simulink model "EPD629_WilliamsJ_Project_20220413_1405"  (R2021b)
settings: Solver=VariableStepAuto  StartTime=0.0  StopTime=25  MaxStep=0.005  RelTol=1e-3
values from neighbouring files (symbols this model uses):
  AxleRatio = 11.47    [ProjectScript.m]
  BrakeDrag_N = 2.5    [ProjectScript.m]
  CableStrokeVsPedalPos_mmpdeg = 0.995519    [ProjectScript.m]
  Cd = 0.7691142    [ProjectScript.m]
  Crr = 0.0138796    [ProjectScript.m]
  CTireRollRadius = 0.944    [ProjectScript.m]
  CVTEff = 0.35    [ProjectScript.m]
  CVTEngagementSpd_rpm = 1400    [ProjectScript.m]
  CVTRatioCoeffVsMphA = 0.000494471902965804    (= 0.000494471902966)    [ProjectScript.m]
  CVTRatioCoeffVsMphB = -0.0203171948865201    (= -0.0203171948865)    [ProjectScript.m]
  CVTRatioCoeffVsMphC = 0.301637634575451    (= 0.301637634575)    [ProjectScript.m]
  CVTRatioCoeffVsMphD = -2.09463337350964    (= -2.09463337351)    [ProjectScript.m]
  CVTRatioCoeffVsMphE = 7.47628950179633    (= 7.4762895018)    [ProjectScript.m]
  DistCableSinkThrottle_mm = 0.25    [ProjectScript.m]
  EngPowerTableData_hp = [0, 0, 0, 0, 0 ... (first row only)    [ProjectScript.m]
  EngPowerTableSpdBreakpoints_rpm = (0:500:7500)    [ProjectScript.m]
  EngPowerTableThrottleBreakpoints_prcnt = [0:.25:1]    [ProjectScript.m]
  FlyCoeffAClosed = 5.31512605042017e-8    (= 5.31512605042e-08)    [ProjectScript.m]
  FlyCoeffAOpen = 2.27450980392157e-7    (= 2.27450980392e-07)    [ProjectScript.m]
  FlyCoeffBClosed = 0.0000162815126050419    (= 1.6281512605e-05)    [ProjectScript.m]
  FlyCoeffBOpen = -0.000070868347338936    (= -7.08683473389e-05)    [ProjectScript.m]
  FlyCoeffCClosed = -0.0102941176470588    (= -0.0102941176471)    [ProjectScript.m]
  FlyCoeffCOpen = 0.00588235294117689    (= 0.00588235294118)    [ProjectScript.m]
  g = 9.80665    [ProjectScript.m]
  GearboxRatio = 1.95    [ProjectScript.m]
  GovArmRange_deg = 14.7    [ProjectScript.m]
  GradeIncline_pcnt = 0    [ProjectScript.m]
  LengthGovArmLower_mm = 90.4    [ProjectScript.m]
  LengthGovArmUpper_mm = 67.5    [ProjectScript.m]
  MassVehicle_kg = (CurbWeight_lbm + VehiclePayload_lbm)*0.4535924    (= 589.67012)    [ProjectScript.m]
  PedalPosMax_deg = 30    [ProjectScript.m]
  PedalTravelIntTension_deg = 10    [ProjectScript.m]
  rho_air = 1.224991    [ProjectScript.m]
  SpringRate_lbfpin = 12.6    [ProjectScript.m]
  ThrottleCableDia_mm = 1.190625    [ProjectScript.m]
  ThrottleLeverArmRadius_mm = 14.25    [ProjectScript.m]
  ThrottlePosMax_deg = 82    [ProjectScript.m]
  ThrottleReturnSpringPreload_Nmm = 163.7711    [ProjectScript.m]
  ThrottleReturnSpringRate_Nmmpdeg = 0.786881    [ProjectScript.m]
  TireDia_in = 18    [ProjectScript.m]
  VehicleFrontalArea_m2 = 1.8    [ProjectScript.m]
libraries: simulink_extras x2
settings Model: Creator=jwilli42  LastModifiedBy=jwilli42

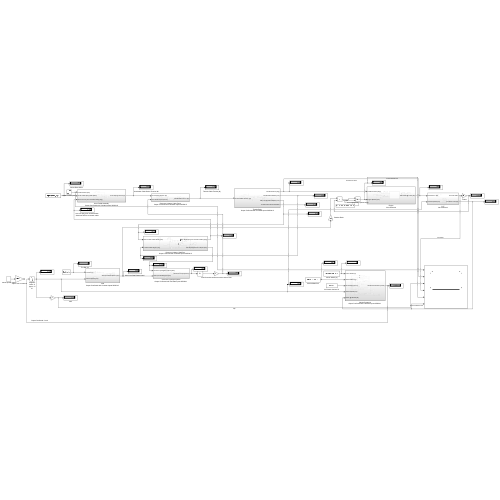
[thumbnail: Simulink's stored preview of the top-level diagram]
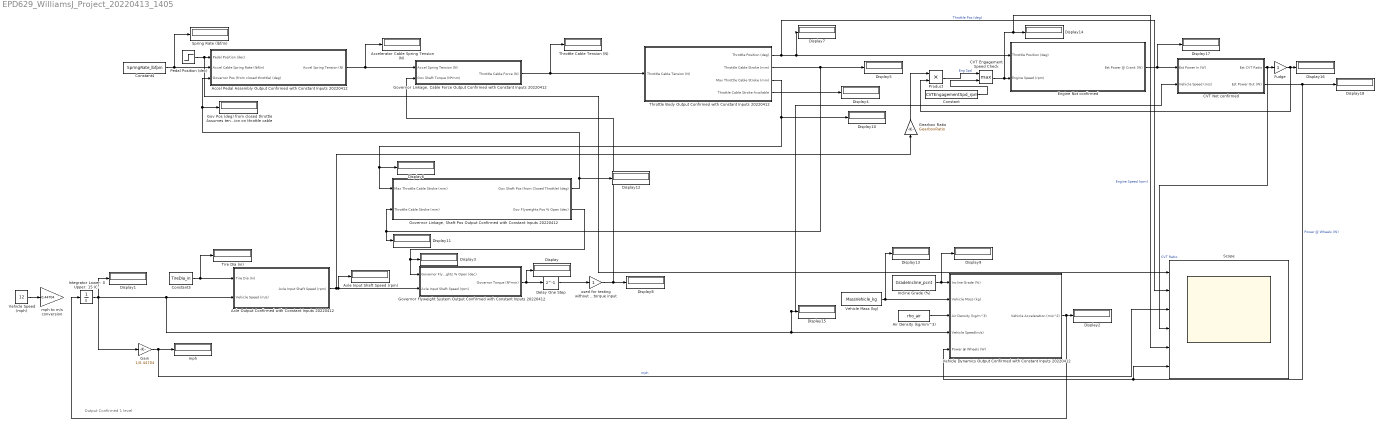
== system EPD629_WilliamsJ_Project_20220413_1405 ==
  note: Output Confirmed 1 level
  Accel Pedal Assembly Output Confirmed with Constant Inputs 20220412 : Subsystem
  Accelerator Cable Spring Tension (N) : Display
  Air Density (kg/mm^3) : Constant  Value=rho_air
  Axle Output Confirmed with Constant Inputs 20220412 : Subsystem
  Axle Input Shaft Speed (rpm) : Display
  CVT Not confirmed : Subsystem
  CVT Engagement Speed Check : MinMax  Function=max  Inputs=2
  Constant : Constant  Value=CVTEngagementSpd_rpm
  Constant3 : Constant  Value=TireDia_in
  Constant4 : Constant  Value=SpringRate_lbfpin
  Delay One Step : Delay  DelayLength=1
  Display{,1..18} (19 alike) : Display
  Engine Not confirmed : Subsystem
  Fudge : Gain
  Gain : Gain  Gain=1/0.44704
  Gearbox Ratio : Gain  Gain=GearboxRatio
  Gov Pos (deg) from closed throttle Assumes tension on throttle cable : Display
  Governor Flyweight System Output Confirmed with Constant Inputs 20220412 : Subsystem
  "Governor Linkage, Cable Force Output Confirmed with Constant Inputs 20220412" : Subsystem
  "Governor Linkage, Shaft Pos Output Confirmed with Constant Inputs 20220412" : Subsystem
  Incline Grade (%) : Constant  Value=GradeIncline_pcnt
  "Integrator Lower: 0 Upper: 15 IC: " : Integrator  InitialCondition=0.1  LimitOutput=on  UpperSaturationLimit=15  LowerSaturationLimit=0
  Pedal Position (dec) : Step  Time=0.5  SampleTime=0
  Product : Product
  Scope : Scope  NumInputPorts=6
  Spring Rate (lbf/in) : Display
  Throttle Body Output Confirmed with Constant Inputs 20220412 : Subsystem
  "Throttle Cable Tension (N) " : Display
  Tire Dia (in) : Display
  "Vehicle Dynamics Output Confirmed with Constant Inputs 20220412 " : Subsystem
  Vehicle Mass (kg) : Constant  Value=MassVehicle_kg
  Vehicle Speed (mph) : Constant  Value=12
  mph : Display
  mph to m/s conversion : Gain  Gain=0.44704
  used for testing without governor torque input : Gain
  wires:
  Incline Grade (%)/1 -> Display9/1, "Vehicle Dynamics Output Confirmed with Constant Inputs 20220412 "/1(Incline Grade (%))
  Vehicle Mass (kg)/1 -> "Vehicle Dynamics Output Confirmed with Constant Inputs 20220412 "/2(Vehicle Mass (kg)), Display13/1
  Air Density (kg/mm^3)/1 -> "Vehicle Dynamics Output Confirmed with Constant Inputs 20220412 "/3(Air Density (kg/m^3))
  "Governor Linkage, Shaft Pos Output Confirmed with Constant Inputs 20220412"/2(Gov Flyweights Pos % Open (dec)) -> Governor Flyweight System Output Confirmed with Constant Inputs 20220412/1(Governor Flyweights % Open (dec)), Display3/1
  Vehicle Speed (mph)/1 -> mph to m/s conversion/1
  Constant3/1 -> Tire Dia (in)/1, Axle Output Confirmed with Constant Inputs 20220412/1(Tire Dia (In))
  Throttle Body Output Confirmed with Constant Inputs 20220412/3(Max Throttle Cable Stroke (mm)) -> Display10/1, "Governor Linkage, Shaft Pos Output Confirmed with Constant Inputs 20220412"/1(Max Throttle Cable Stroke (mm)), Display6/1
  Axle Output Confirmed with Constant Inputs 20220412/1(Axle Input Shaft Speed (rpm)) -> Governor Flyweight System Output Confirmed with Constant Inputs 20220412/2(Axle Input Shaft Speed (rpm)), Axle Input Shaft Speed (rpm)/1, Gearbox Ratio/1
  Accel Pedal Assembly Output Confirmed with Constant Inputs 20220412/1(Accel Spring Tension (N)) -> Accelerator Cable Spring Tension (N)/1, "Governor Linkage, Cable Force Output Confirmed with Constant Inputs 20220412"/1(Accel Spring Tension (N))
  Constant4/1 -> Spring Rate (lbf/in)/1, Accel Pedal Assembly Output Confirmed with Constant Inputs 20220412/2(Accel Cable Spring Rate (lbf/in))
  Pedal Position (dec)/1 -> Scope/1, Accel Pedal Assembly Output Confirmed with Constant Inputs 20220412/1(Pedal Position (dec))
  Throttle Body Output Confirmed with Constant Inputs 20220412/1(Throttle Position (deg)) -> Scope/2, Engine Not confirmed/1(Throttle Position (deg)), Display7/1  "Throttle Pos (deg)"
  Governor Flyweight System Output Confirmed with Constant Inputs 20220412/1(Governor Torque (N*mm)) -> Delay One Step/1, Display/1
  "Governor Linkage, Shaft Pos Output Confirmed with Constant Inputs 20220412"/1(Gov Shaft Pos (from Closed Throttle) (deg)) -> Accel Pedal Assembly Output Confirmed with Constant Inputs 20220412/3(Governor Pos (from closed throttle) (deg)), Gov Pos (deg) from closed throttle Assumes tension on throttle cable/1, Display12/1
  used for testing without governor torque input/1 -> Display8/1, "Governor Linkage, Cable Force Output Confirmed with Constant Inputs 20220412"/2(Gov Shaft Torque (N*mm))
  "Governor Linkage, Cable Force Output Confirmed with Constant Inputs 20220412"/1(Throttle Cable Force (N)) -> "Throttle Cable Tension (N) "/1, Throttle Body Output Confirmed with Constant Inputs 20220412/1(Throttle Cable Tension (N))
  Throttle Body Output Confirmed with Constant Inputs 20220412/4(Throttle Cable Stroke Available) -> Display4/1
  Throttle Body Output Confirmed with Constant Inputs 20220412/2(Throttle Cable Stroke (mm)) -> "Governor Linkage, Shaft Pos Output Confirmed with Constant Inputs 20220412"/2(Throttle Cable Stroke (mm)), Display11/1, Display5/1
  "Vehicle Dynamics Output Confirmed with Constant Inputs 20220412 "/1(Vehicle Acceleration (m/s^2)) -> "Integrator Lower: 0 Upper: 15 IC: "/1, Display2/1
  Engine Not confirmed/1(Est Power @ Crank (W)) -> Display17/1, CVT Not confirmed/1(Est Power In (W))
  Gearbox Ratio/1 -> Product/1
  CVT Not confirmed/1(Est CVT Ratio) -> Scope/4, Fudge/1  "CVT Ratio"
  Fudge/1 -> Display16/1, Product/2
  CVT Not confirmed/2(Est Power Out (W)) -> Scope/6, "Vehicle Dynamics Output Confirmed with Constant Inputs 20220412 "/5(Power @ Wheels (W)), Display18/1  "Power @ Wheels (W)"
  "Integrator Lower: 0 Upper: 15 IC: "/1 -> Gain/1, Display15/1, CVT Not confirmed/2(Vehicle Speed (m/s)), "Vehicle Dynamics Output Confirmed with Constant Inputs 20220412 "/4(Vehicle Speed(m/s)), Axle Output Confirmed with Constant Inputs 20220412/2(Vehicle Speed (m/s)), Display1/1
  Gain/1 -> Scope/3, mph/1  "mph"
  Product/1 -> CVT Engagement Speed Check/1  "Eng Spd"
  Constant/1 -> CVT Engagement Speed Check/2
  Delay One Step/1 -> used for testing without governor torque input/1
  CVT Engagement Speed Check/1 -> Scope/5, Display14/1, Engine Not confirmed/2(Engine Speed (rpm))  "Engine Speed (rpm)"

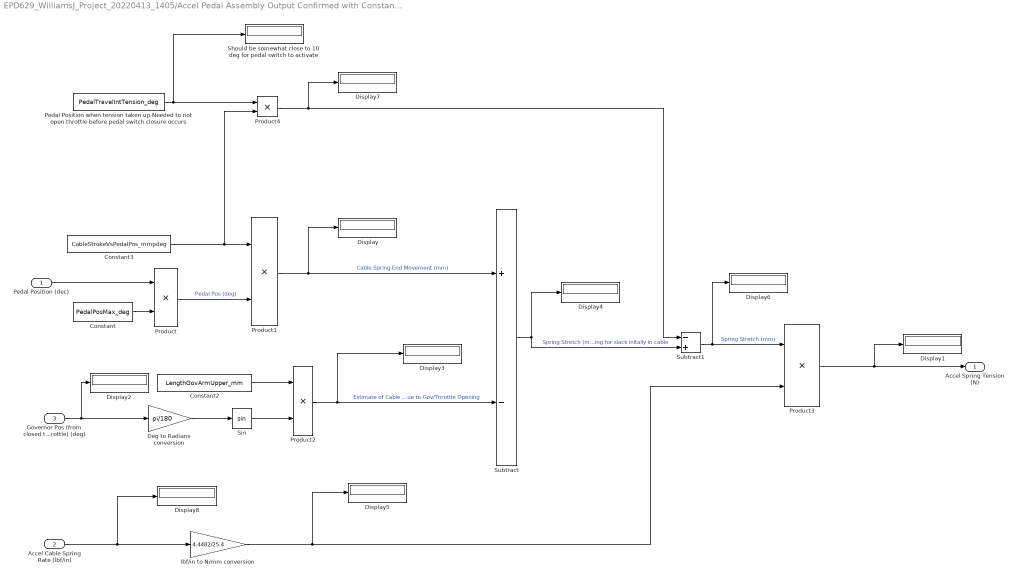
== system EPD629_WilliamsJ_Project_20220413_1405/Accel Pedal Assembly Output Confirmed with Constant Inputs 20220412 ==
  Pedal Position (dec) : Inport
  Accel Cable Spring Rate (lbf/in) : Inport  Port=2
  Governor Pos (from closed throttle) (deg) : Inport  Port=3
  Constant : Constant  Value=PedalPosMax_deg
  Constant2 : Constant  Value=LengthGovArmUpper_mm
  Constant3 : Constant  Value=CableStrokeVsPedalPos_mmpdeg
  Deg to Radians conversion : Gain  Gain=pi/180
  Display{,1..8} (9 alike) : Display
  Pedal Position when tension taken up Needed to not open throttle before pedal switch closure occurs : Constant  Value=PedalTravelIntTension_deg
  Product{,1..4} (5 alike) : Product
  Should be somewhat close to 10 deg for pedal switch to activate : Display
  Sin : Trigonometry
  Subtract : Sum  Inputs=+-
  Subtract1 : Sum  Inputs=-+
  lbf/in to N/mm conversion : Gain  Gain=4.4482/25.4
  Accel Spring Tension (N) : Outport
  wires:
  Constant/1 -> Product/2
  Product/1 -> Product1/2  "Pedal Pos (deg)"
  Governor Pos (from closed throttle) (deg)/1 -> Display2/1, Deg to Radians conversion/1
  Deg to Radians conversion/1 -> Sin/1
  Sin/1 -> Product2/2
  Constant2/1 -> Product2/1
  Product1/1 -> Display/1, Subtract/1  "Cable Spring End Movement (mm)"
  Product2/1 -> Display3/1, Subtract/2  "Estimate of Cable Travel Due to Gov/Throttle Opening"
  lbf/in to N/mm conversion/1 -> Display5/1, Product3/2
  Subtract/1 -> Subtract1/2, Display4/1  "Spring Stretch (mm) w/out accounting for slack initally in cable"
  Product3/1 -> Display1/1, Accel Spring Tension (N)/1
  Accel Cable Spring Rate (lbf/in)/1 -> Display8/1, lbf/in to N/mm conversion/1
  Product4/1 -> Subtract1/1, Display7/1
  Subtract1/1 -> Display6/1, Product3/1  "Spring Stretch (mm)"
  Pedal Position (dec)/1 -> Product/1
  Pedal Position when tension taken up Needed to not open throttle before pedal switch closure occurs/1 -> Should be somewhat close to 10 deg for pedal switch to activate/1, Product4/1
  Constant3/1 -> Product1/1, Product4/2

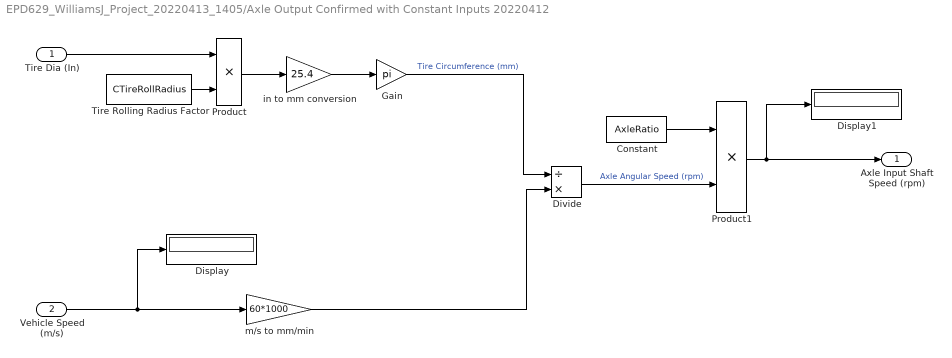
== system EPD629_WilliamsJ_Project_20220413_1405/Axle Output Confirmed with Constant Inputs 20220412 ==
  Tire Dia (In) : Inport
  Vehicle Speed (m/s) : Inport  Port=2
  Constant : Constant  Value=AxleRatio
  Display : Display
  Display1 : Display
  Divide : Product  Inputs=/*
  Gain : Gain  Gain=pi
  Product : Product
  Product1 : Product
  Tire Rolling Radius Factor : Constant  Value=CTireRollRadius
  in to mm conversion : Gain  Gain=25.4
  m/s to mm/min : Gain  Gain=60*1000
  Axle Input Shaft Speed (rpm) : Outport
  wires:
  Tire Rolling Radius Factor/1 -> Product/2
  Tire Dia (In)/1 -> Product/1
  Product/1 -> in to mm conversion/1
  in to mm conversion/1 -> Gain/1
  Gain/1 -> Divide/1  "Tire Circumference (mm)"
  Vehicle Speed (m/s)/1 -> Display/1, m/s to mm/min/1
  m/s to mm/min/1 -> Divide/2
  Divide/1 -> Product1/2  "Axle Angular Speed (rpm)"
  Constant/1 -> Product1/1
  Product1/1 -> Display1/1, Axle Input Shaft Speed (rpm)/1

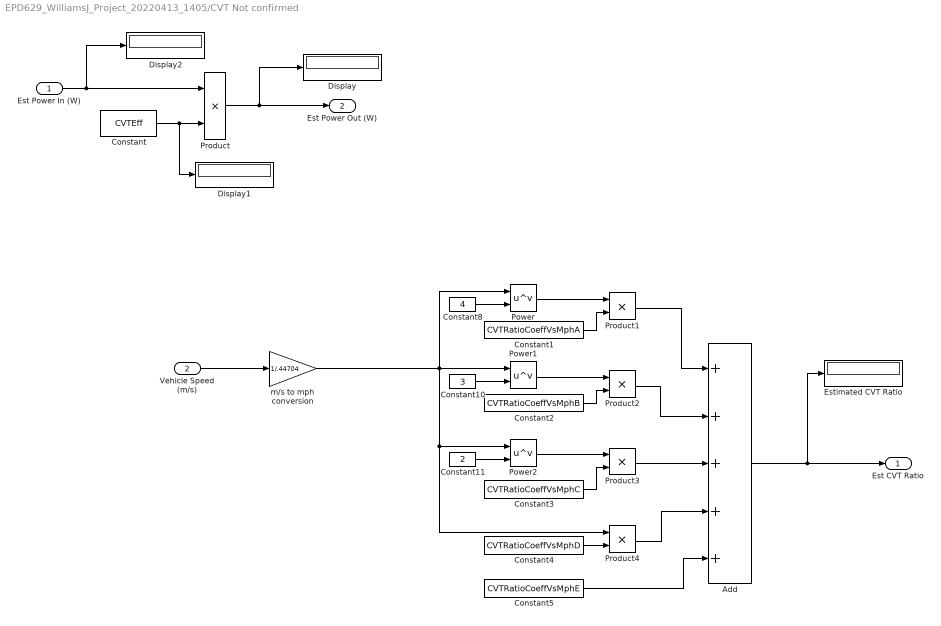
== system EPD629_WilliamsJ_Project_20220413_1405/CVT Not confirmed ==
  Est Power In (W) : Inport
  Vehicle Speed (m/s) : Inport  Port=2
  Add : Sum  Inputs=+++++
  Constant : Constant  Value=CVTEff
  Constant1 : Constant  Value=CVTRatioCoeffVsMphA
  Constant10 : Constant  Value=3
  Constant11 : Constant  Value=2
  Constant2 : Constant  Value=CVTRatioCoeffVsMphB
  Constant3 : Constant  Value=CVTRatioCoeffVsMphC
  Constant4 : Constant  Value=CVTRatioCoeffVsMphD
  Constant5 : Constant  Value=CVTRatioCoeffVsMphE
  Constant8 : Constant  Value=4
  Display : Display
  Display1 : Display
  Display2 : Display
  Estimated CVT Ratio : Display
  Power : Math  Operator=pow  SaturateOnIntegerOverflow=on
  Power1 : Math  Operator=pow  SaturateOnIntegerOverflow=on
  Power2 : Math  Operator=pow  SaturateOnIntegerOverflow=on
  Product{,1..4} (5 alike) : Product
  m/s to mph conversion : Gain  Gain=1/.44704
  Est CVT Ratio : Outport
  Est Power Out (W) : Outport  Port=2
  wires:
  Est Power In (W)/1 -> Display2/1, Product/1
  Constant/1 -> Product/2, Display1/1
  Product/1 -> Display/1, Est Power Out (W)/1
  Constant8/1 -> Power/2
  Power/1 -> Product1/1
  Constant1/1 -> Product1/2
  Constant10/1 -> Power1/2
  Constant11/1 -> Power2/2
  m/s to mph conversion/1 -> Power/1, Product4/1, Power2/1, Power1/1
  Power1/1 -> Product2/1
  Constant2/1 -> Product2/2
  Power2/1 -> Product3/1
  Constant3/1 -> Product3/2
  Constant4/1 -> Product4/2
  Product3/1 -> Add/3
  Product2/1 -> Add/2
  Product1/1 -> Add/1
  Product4/1 -> Add/4
  Constant5/1 -> Add/5
  Add/1 -> Estimated CVT Ratio/1, Est CVT Ratio/1
  Vehicle Speed (m/s)/1 -> m/s to mph conversion/1

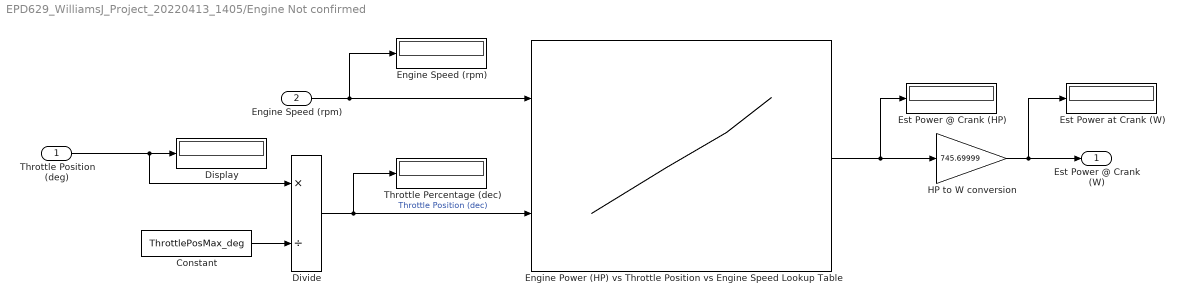
== system EPD629_WilliamsJ_Project_20220413_1405/Engine Not confirmed ==
  Throttle Position (deg) : Inport
  Engine Speed (rpm) : Inport  Port=2
  Constant : Constant  Value=ThrottlePosMax_deg
  Display : Display
  Divide : Product  Inputs=*/
  Engine Power (HP) vs Throttle Position vs Engine Speed Lookup Table : Lookup_n-D  BreakpointsForDimension1=EngPowerTableSpdBreakpoints_rpm  BreakpointsForDimension2=EngPowerTableThrottleBreakpoints_prcnt  Table=EngPowerTableData_hp  InternalRulePriority=Speed  RndMeth=Simplest  InputSameDT=on
      settings: InputPortMap=u0,u1
  "Engine Speed (rpm) " : Display
  Est Power @ Crank (HP) : Display
  Est Power at Crank (W) : Display
  HP to W conversion : Gain  Gain=745.69999
  Throttle Percentage (dec) : Display
  Est Power @ Crank (W) : Outport
  wires:
  Constant/1 -> Divide/2
  Divide/1 -> Engine Power (HP) vs Throttle Position vs Engine Speed Lookup Table/2, Throttle Percentage (dec)/1  "Throttle Position (dec)"
  Throttle Position (deg)/1 -> Display/1, Divide/1
  Engine Power (HP) vs Throttle Position vs Engine Speed Lookup Table/1 -> Est Power @ Crank (HP)/1, HP to W conversion/1
  HP to W conversion/1 -> Est Power at Crank (W)/1, Est Power @ Crank (W)/1
  Engine Speed (rpm)/1 -> "Engine Speed (rpm) "/1, Engine Power (HP) vs Throttle Position vs Engine Speed Lookup Table/1

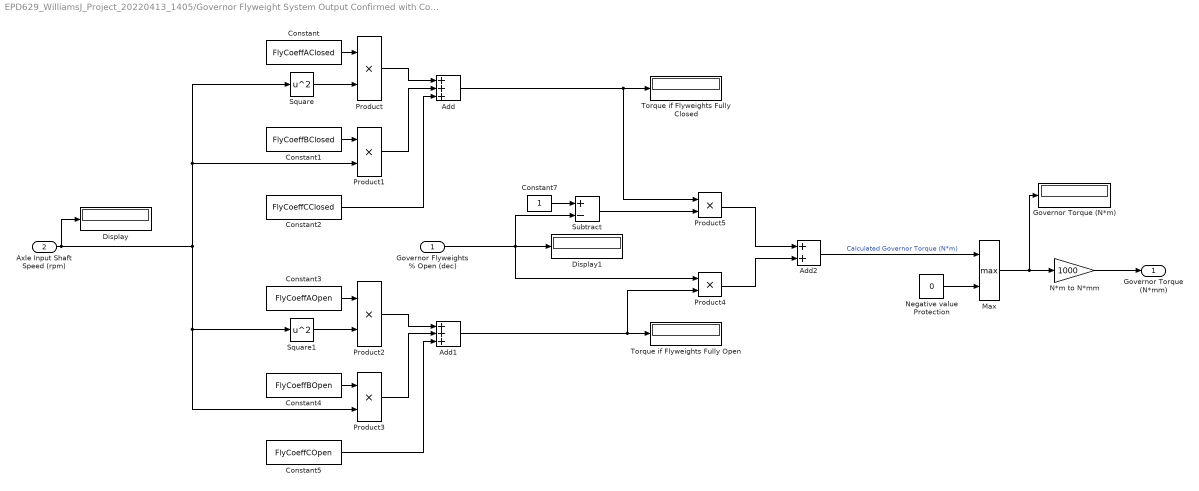
== system EPD629_WilliamsJ_Project_20220413_1405/Governor Flyweight System Output Confirmed with Constant Inputs 20220412 ==
  Governor Flyweights % Open (dec) : Inport
  Axle Input Shaft Speed (rpm) : Inport  Port=2
  Add : Sum  Inputs=+++
  Add1 : Sum  Inputs=+++
  Add2 : Sum
  Constant : Constant  Value=FlyCoeffAClosed
  Constant1 : Constant  Value=FlyCoeffBClosed
  Constant2 : Constant  Value=FlyCoeffCClosed
  Constant3 : Constant  Value=FlyCoeffAOpen
  Constant4 : Constant  Value=FlyCoeffBOpen
  Constant5 : Constant  Value=FlyCoeffCOpen
  Constant7 : Constant
  Display : Display
  Display1 : Display
  Governor Torque (N*m) : Display
  Max : MinMax  Function=max  Inputs=2
  N*m to N*mm : Gain  Gain=1000
  Negative value Protection : Constant  Value=0
  Product{,1..5} (6 alike) : Product
  Square : Math  Operator=square  SaturateOnIntegerOverflow=on
  Square1 : Math  Operator=square  SaturateOnIntegerOverflow=on
  Subtract : Sum  Inputs=+-
  Torque if Flyweights Fully Closed : Display
  Torque if Flyweights Fully Open : Display
  Governor Torque (N*mm) : Outport
  wires:
  Axle Input Shaft Speed (rpm)/1 -> Product1/2, Square/1, Square1/1, Product3/2, Display/1
  Product/1 -> Add/1
  Product1/1 -> Add/2
  Constant2/1 -> Add/3
  Constant1/1 -> Product1/1
  Constant/1 -> Product/1
  Square/1 -> Product/2
  Square1/1 -> Product2/2
  Constant3/1 -> Product2/1
  Constant4/1 -> Product3/1
  Constant5/1 -> Add1/3
  Product3/1 -> Add1/2
  Product2/1 -> Add1/1
  N*m to N*mm/1 -> Governor Torque (N*mm)/1
  Negative value Protection/1 -> Max/2
  Max/1 -> Governor Torque (N*m)/1, N*m to N*mm/1
  Add2/1 -> Max/1  "Calculated Governor Torque (N*m)"
  Constant7/1 -> Subtract/1
  Governor Flyweights % Open (dec)/1 -> Display1/1, Subtract/2, Product4/1
  Add1/1 -> Torque if Flyweights Fully Open/1, Product4/2
  Product4/1 -> Add2/2
  Subtract/1 -> Product5/2
  Add/1 -> Torque if Flyweights Fully Closed/1, Product5/1
  Product5/1 -> Add2/1

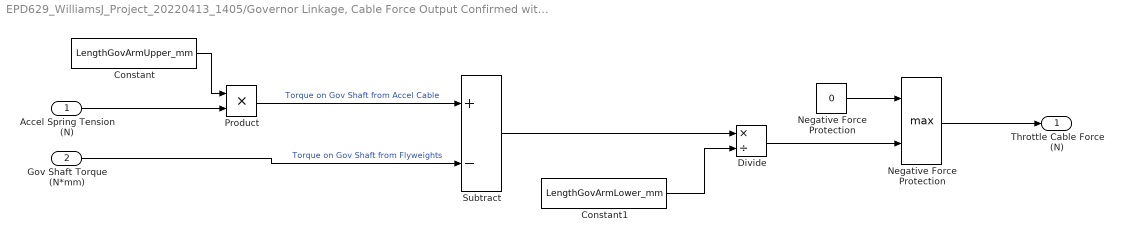
== system EPD629_WilliamsJ_Project_20220413_1405/Governor Linkage, Cable Force Output Confirmed with Constant Inputs 20220412 ==
  Accel Spring Tension (N) : Inport
  Gov Shaft Torque (N*mm) : Inport  Port=2
  Constant : Constant  Value=LengthGovArmUpper_mm
  Constant1 : Constant  Value=LengthGovArmLower_mm
  Divide : Product  Inputs=*/
  Negative Force Protection : Constant  Value=0
  "Negative Force Protection " : MinMax  Function=max  Inputs=2
  Product : Product
  Subtract : Sum  Inputs=+-
  Throttle Cable Force (N) : Outport
  wires:
  Accel Spring Tension (N)/1 -> Product/2
  Constant/1 -> Product/1
  Product/1 -> Subtract/1  "Torque on Gov Shaft from Accel Cable"
  Gov Shaft Torque (N*mm)/1 -> Subtract/2  "Torque on Gov Shaft from Flyweights"
  Subtract/1 -> Divide/1
  Constant1/1 -> Divide/2
  Divide/1 -> "Negative Force Protection "/2
  Negative Force Protection/1 -> "Negative Force Protection "/1
  "Negative Force Protection "/1 -> Throttle Cable Force (N)/1

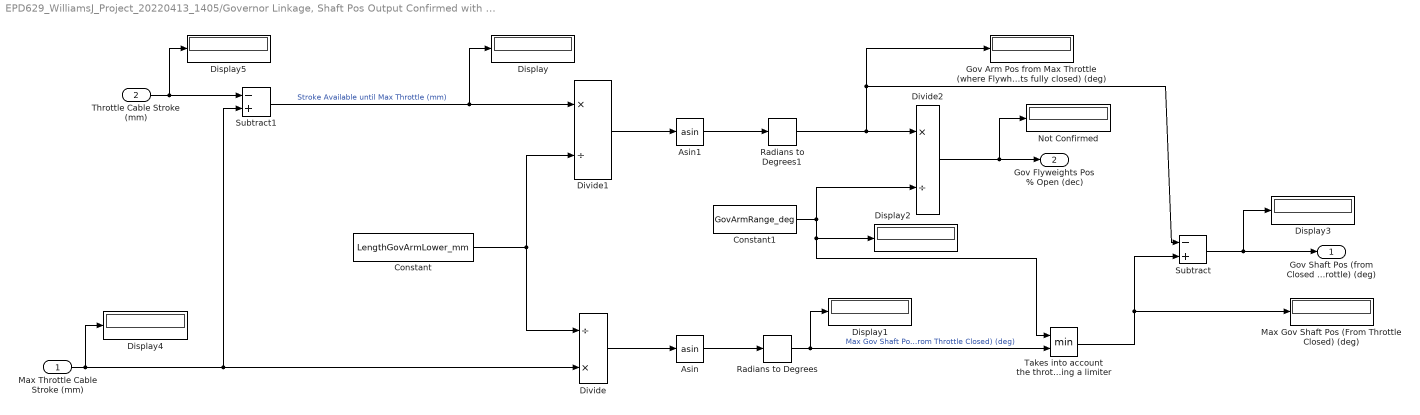
== system EPD629_WilliamsJ_Project_20220413_1405/Governor Linkage, Shaft Pos Output Confirmed with Constant Inputs 20220412 ==
  Max Throttle Cable Stroke (mm) : Inport
  Throttle Cable Stroke (mm) : Inport  Port=2
  Asin : Trigonometry  Operator=asin
  Asin1 : Trigonometry  Operator=asin
  Constant : Constant  Value=LengthGovArmLower_mm
  Constant1 : Constant  Value=GovArmRange_deg
  Display{,1..5} (6 alike) : Display
  Divide : Product  Inputs=/*
  Divide1 : Product  Inputs=*/
  Divide2 : Product  Inputs=*/
  Gov Arm Pos from Max Throttle (where Flywheights fully closed) (deg) : Display
  Max Gov Shaft Pos (From Throttle Closed) (deg) : Display
  Not Confirmed : Display
  Radians to Degrees : simulink_extras/Transformations/Radians to Degrees
  Radians to Degrees1 : simulink_extras/Transformations/Radians to Degrees
  Subtract : Sum  Inputs=-+
  Subtract1 : Sum  Inputs=-+
  Takes into account the throttle stop OR the governor shaft stop being a limiter : MinMax  Inputs=2
  Gov Shaft Pos (from Closed Throttle) (deg) : Outport
  Gov Flyweights Pos % Open (dec) : Outport  Port=2
  wires:
  Max Throttle Cable Stroke (mm)/1 -> Display4/1, Subtract1/2, Divide/2
  Divide/1 -> Asin/1
  Asin/1 -> Radians to Degrees/1
  Radians to Degrees/1 -> Takes into account the throttle stop OR the governor shaft stop being a limiter/2, Display1/1  "Max Gov Shaft Pos (From Throttle Closed) (deg)"
  Constant/1 -> Divide1/2, Divide/1
  Divide1/1 -> Asin1/1
  Asin1/1 -> Radians to Degrees1/1
  Radians to Degrees1/1 -> Gov Arm Pos from Max Throttle (where Flywheights fully closed) (deg)/1, Subtract/1, Divide2/1
  Divide2/1 -> Not Confirmed/1, Gov Flyweights Pos % Open (dec)/1
  Constant1/1 -> Divide2/2, Display2/1, Takes into account the throttle stop OR the governor shaft stop being a limiter/1
  Takes into account the throttle stop OR the governor shaft stop being a limiter/1 -> Subtract/2, Max Gov Shaft Pos (From Throttle Closed) (deg)/1
  Subtract/1 -> Display3/1, Gov Shaft Pos (from Closed Throttle) (deg)/1
  Subtract1/1 -> Divide1/1, Display/1  "Stroke Available until Max Throttle (mm)"
  Throttle Cable Stroke (mm)/1 -> Subtract1/1, Display5/1

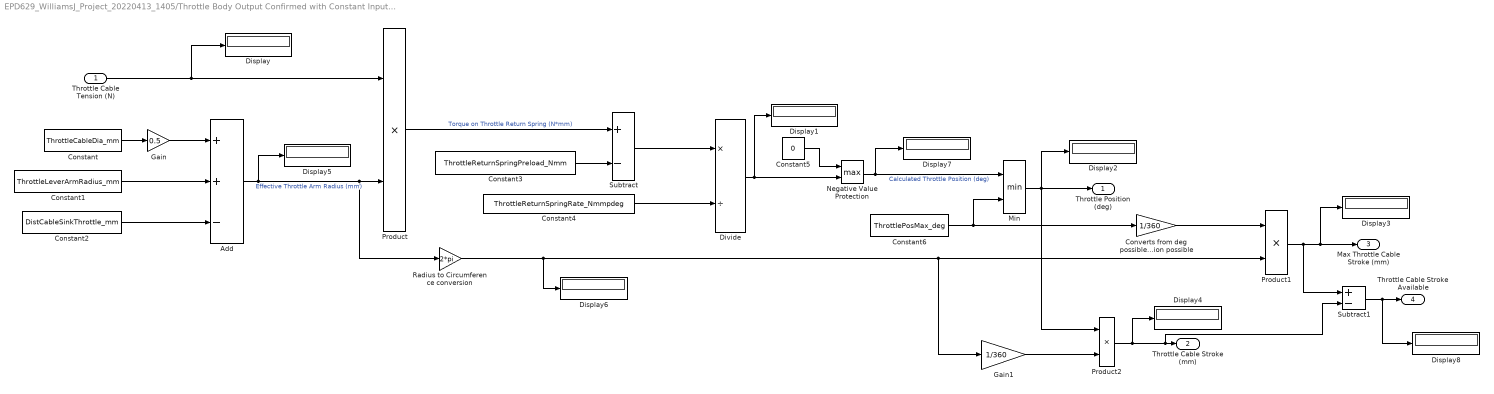
== system EPD629_WilliamsJ_Project_20220413_1405/Throttle Body Output Confirmed with Constant Inputs 20220412 ==
  Throttle Cable Tension (N) : Inport
  Add : Sum  Inputs=++-
  Constant : Constant  Value=ThrottleCableDia_mm
  Constant1 : Constant  Value=ThrottleLeverArmRadius_mm
  Constant2 : Constant  Value=DistCableSinkThrottle_mm
  Constant3 : Constant  Value=ThrottleReturnSpringPreload_Nmm
  Constant4 : Constant  Value=ThrottleReturnSpringRate_Nmmpdeg
  Constant5 : Constant  Value=0
  Constant6 : Constant  Value=ThrottlePosMax_deg
  Converts from deg possible to percentage of rotation possible : Gain  Gain=1/360
  Display{,1..8} (9 alike) : Display
  Divide : Product  Inputs=*/
  Gain : Gain  Gain=0.5
  Gain1 : Gain  Gain=1/360
  Min : MinMax  Inputs=2
  Negative Value Protection : MinMax  Function=max  Inputs=2
  Product : Product
  Product1 : Product
  Product2 : Product
  Radius to Circumference conversion : Gain  Gain=2*pi
  Subtract : Sum  Inputs=+-
  Subtract1 : Sum  Inputs=+-
  Throttle Position (deg) : Outport
  Throttle Cable Stroke (mm) : Outport  Port=2
  Max Throttle Cable Stroke (mm) : Outport  Port=3
  Throttle Cable Stroke Available : Outport  Port=4
  wires:
  Constant/1 -> Gain/1
  Gain/1 -> Add/1
  Constant1/1 -> Add/2
  Constant2/1 -> Add/3
  Add/1 -> Display5/1, Product/2, Radius to Circumference conversion/1  "Effective Throttle Arm Radius (mm)"
  Product/1 -> Subtract/1  "Torque on Throttle Return Spring (N*mm)"
  Constant3/1 -> Subtract/2
  Subtract/1 -> Divide/1
  Constant4/1 -> Divide/2
  Constant5/1 -> Negative Value Protection/1
  Divide/1 -> Display1/1, Negative Value Protection/2
  Negative Value Protection/1 -> Display7/1, Min/1  "Calculated Throttle Position (deg)"
  Constant6/1 -> Min/2, Converts from deg possible to percentage of rotation possible/1
  Min/1 -> Display2/1, Throttle Position (deg)/1, Product2/1
  Converts from deg possible to percentage of rotation possible/1 -> Product1/1
  Radius to Circumference conversion/1 -> Product1/2, Gain1/1, Display6/1
  Product1/1 -> Display3/1, Max Throttle Cable Stroke (mm)/1, Subtract1/1
  Product2/1 -> Display4/1, Subtract1/2, Throttle Cable Stroke (mm)/1
  Gain1/1 -> Product2/2
  Throttle Cable Tension (N)/1 -> Display/1, Product/1
  Subtract1/1 -> Display8/1, Throttle Cable Stroke Available/1

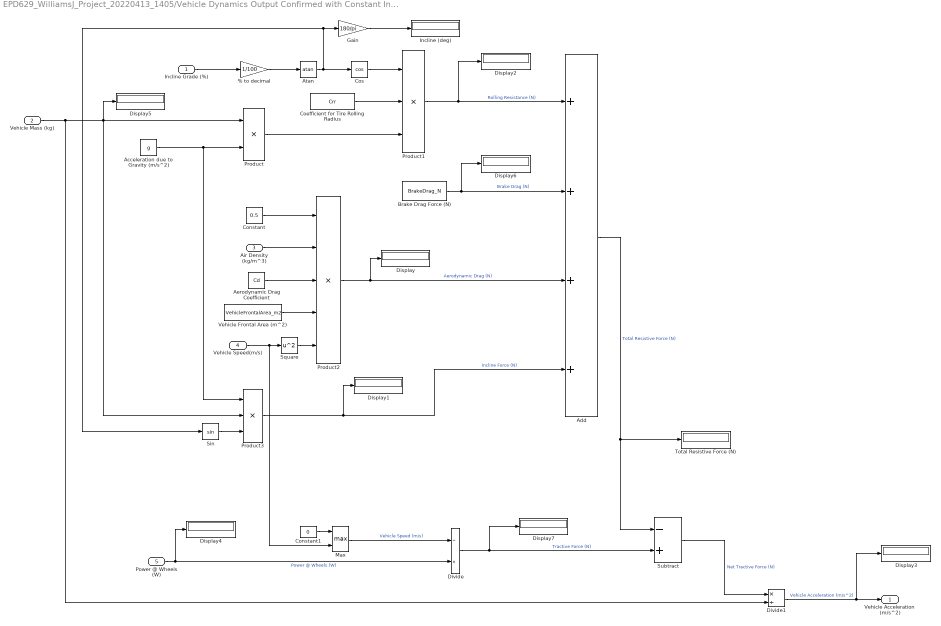
== system EPD629_WilliamsJ_Project_20220413_1405/Vehicle Dynamics Output Confirmed with Constant Inputs 20220412  ==
  Incline Grade (%) : Inport
  Vehicle Mass (kg) : Inport  Port=2
  Air Density (kg/m^3) : Inport  Port=3
  Vehicle Speed(m/s) : Inport  Port=4
  Power @ Wheels (W) : Inport  Port=5
  % to decimal : Gain  Gain=1/100
  Acceleration due to Gravity (m/s^2) : Constant  Value=g
  Add : Sum  Inputs=++++
  Aerodynamic Drag Coefficient : Constant  Value=Cd
  Atan : Trigonometry  Operator=atan
  Brake Drag Force (N) : Constant  Value=BrakeDrag_N
  Coefficient for Tire Rolling Radius : Constant  Value=Crr
  Constant : Constant  Value=0.5
  Constant1 : Constant  Value=0
  Cos : Trigonometry  Operator=cos
  Display{,1..7} (8 alike) : Display
  Divide : Product  Inputs=/*
  Divide1 : Product  Inputs=*/
  Gain : Gain  Gain=180/pi
  Incline (deg) : Display
  Max : MinMax  Function=max  Inputs=2
  Product : Product
  Product1 : Product  Inputs=3
  Product2 : Product  Inputs=5
  Product3 : Product  Inputs=3
  Sin : Trigonometry
  Square : Math  Operator=square  SaturateOnIntegerOverflow=on
  Subtract : Sum  Inputs=-+
  Total Resistive Force (N) : Display
  Vehicle Frontal Area (m^2) : Constant  Value=VehicleFrontalArea_m2
  Vehicle Acceleration (m/s^2) : Outport
  wires:
  Incline Grade (%)/1 -> % to decimal/1
  % to decimal/1 -> Atan/1
  Gain/1 -> Incline (deg)/1
  Atan/1 -> Sin/1, Gain/1, Cos/1
  Vehicle Mass (kg)/1 -> Display5/1, Product3/2, Product/1, Divide1/2
  Acceleration due to Gravity (m/s^2)/1 -> Product/2, Product3/1
  Cos/1 -> Product1/1
  Coefficient for Tire Rolling Radius/1 -> Product1/2
  Product/1 -> Product1/3
  Product1/1 -> Display2/1, Add/1  "Rolling Resistance (N)"
  Vehicle Speed(m/s)/1 -> Square/1, Max/2
  Constant/1 -> Product2/1
  Air Density (kg/m^3)/1 -> Product2/2
  Aerodynamic Drag Coefficient/1 -> Product2/3
  Vehicle Frontal Area (m^2)/1 -> Product2/4
  Square/1 -> Product2/5
  Product2/1 -> Add/3, Display/1  "Aerodynamic Drag (N)"
  Brake Drag Force (N)/1 -> Display6/1, Add/2  "Brake Drag (N)"
  Sin/1 -> Product3/3
  Product3/1 -> Display1/1, Add/4  "Incline Force (N)"
  Add/1 -> Total Resistive Force (N)/1, Subtract/1  "Total Resistive Force (N)"
  Power @ Wheels (W)/1 -> Display4/1, Divide/2  "Power @ Wheels (W)"
  Constant1/1 -> Max/1
  Max/1 -> Divide/1  "Vehicle Speed (m/s)"
  Divide/1 -> Display7/1, Subtract/2  "Tractive Force (N)"
  Subtract/1 -> Divide1/1  "Net Tractive Force (N)"
  Divide1/1 -> Display3/1, Vehicle Acceleration (m/s^2)/1  "Vehicle Acceleration (m/s^2)"
